simulink model "Simulation2"  (R2023b)
settings: Solver=VariableStepAuto  StartTime=0.0  StopTime=2  RelTol=1e-3
settings Model: Creator=vande_2  LastModifiedBy=vande_2

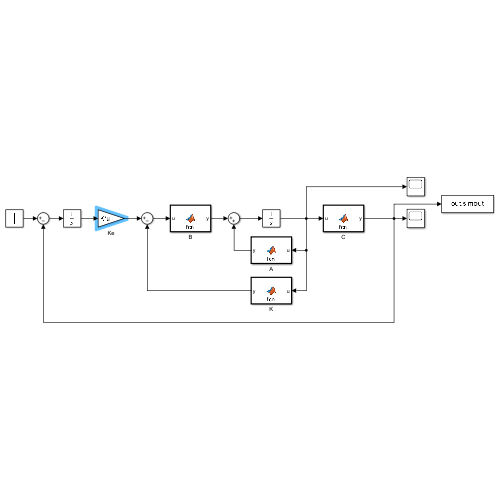
[thumbnail: Simulink's stored preview of the top-level diagram]
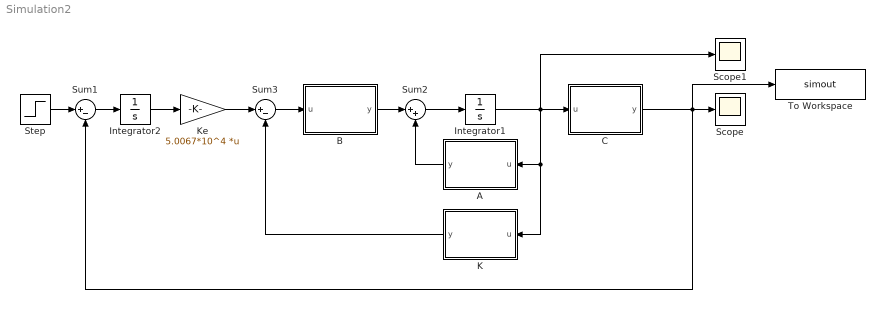
== system Simulation2 ==
  A : MATLAB Function  TreatAsAtomicUnit=on
  B : MATLAB Function  TreatAsAtomicUnit=on
  C : MATLAB Function  TreatAsAtomicUnit=on
  Integrator1 : Integrator
  Integrator2 : Integrator
  K : MATLAB Function  TreatAsAtomicUnit=on
  Ke : Gain  Gain=5.0067*10^4  Multiplication=Matrix(K*u)
  Scope : Scope
  Scope1 : Scope
  Step : Step  Time=0  SampleTime=0
  Sum1 : Sum  Inputs=|+-
  Sum2 : Sum  Inputs=|++
  Sum3 : Sum  Inputs=|+-
  To Workspace : ToWorkspace  VariableName=simout  SaveFormat=Timeseries  SampleTime=-1
  wires:
  Sum3/1 -> B/1(u)
  K/1(y) -> Sum3/2
  Integrator1/1 -> Scope1/1, A/1(u), K/1(u), C/1(u)
  Sum2/1 -> Integrator1/1
  A/1(y) -> Sum2/2
  B/1(y) -> Sum2/1
  Ke/1 -> Sum3/1
  Integrator2/1 -> Ke/1
  Sum1/1 -> Integrator2/1
  Step/1 -> Sum1/1
  C/1(y) -> To Workspace/1, Sum1/2, Scope/1

== matlab function Simulation2/K ==
  data: u input; y output
function y = fcn(u)
K = [418.169 47.4304];
y = K*u;

== matlab function Simulation2/B ==
  data: u input; y output
function y = fcn(u)
B = [0; 1];
y = B*u;

== matlab function Simulation2/C ==
  data: u input; y output
function y = fcn(u)
C = [0.07843, 0];
y = C*u;

== matlab function Simulation2/A ==
  data: u input; y output
function y = fcn(u)
A = [0 1; 0 -0.5696];
y = A*u;
